simulink model "ThdRwRtStFwdBkwdCtrl"  (R2024b)
settings: Solver=FixedStepDiscrete  StartTime=0.0  StopTime=10.0  FixedStep=0.01  RelTol=1e-3
undefined symbols (not defined in the file or in its folder): KeSMSuMdMotFinshdTm_Val, KeSMSuMdRetryTm1_Val, KeSMSuModeReqDurgTm_Val
libraries: StCtrlLibBkRecln x1
settings Model: ModifiedHistory="2024.6.21 V2.1.0  557模式流程V1.6"  Creator=sn2xws  LastModifiedBy=sn55gm
settings SolverCC: AlgebraicLoopSolver=TrustRegion
settings DataIOCC: SaveFormat=StructureWithTime  ReturnWorkspaceOutputs=off
settings OptimizationCC: DefaultParameterBehavior=Inlined  EnhancedBackFolding=on  PassReuseOutputArgsAs=Individual arguments  ZeroExternalMemoryAtStartup=off  ZeroInternalMemoryAtStartup=off  OptimizeBlockOrder=speed  DifferentSizesBufferReuse=on  OptimizationCustomize=off  EfficientTunableParamExpr=on
settings DebuggingCC: ParameterTunabilityLossMsg=error  UnconnectedInputMsg=warning  UnconnectedOutputMsg=warning  UnconnectedLineMsg=warning  ArithmeticOperatorsInVariantConditions=warning
settings ModelReferenceCC: EnableRefExpFcnMdlSchedulingChecks=on  ModelReferenceNumInstancesAllowed=Single
settings SFSimCC: MATLABDynamicMemAlloc=off  CustomCodeUndefinedFunction=UseInterfaceOnly
settings RTWCC: Description=AUTOSAR  SystemTargetFile=autosar.tlc  GenCodeOnly=on  TemplateMakefile=ert_default_tmf  GenerateReport=on  IncludeHyperlinkInReport=on  LaunchReport=on  DataTypeReplacement=CDataTypesFixedWidth  GenerateTraceInfo=on  GenerateTraceReport=on  GenerateTraceReportSl=on  GenerateTraceReportSf=on  GenerateTraceReportEml=on  GPUComputeCapability=3.5
settings CodeAppCC: ForceParamTrailComments=on  IgnoreCustomStorageClasses=off  OperatorAnnotations=on  SimulinkDataObjDesc=on  SFDataObjDesc=on  InsertBlockDesc=on
settings STFCustomTargetCC: TargetLangStandard=C99 (ISO)  MultiwordLength=256  ParMdlRefBuildCompliant=on  CompOptLevelCompliant=on  IncludeMdlTerminateFcn=off  CombineOutputUpdateFcns=on  SuppressErrorStatus=on  ERTCustomFileBanners=on  SupportNonFinite=off  SupportComplex=off  SupportContinuousTime=off  SupportNonInlinedSFcns=off  RemoveResetFunc=on  MATLABClassNameForMDSCustomization=Simulink.SoftwareTarget.ERTCustomization  AutosarCompliant=on  UseToolchainInfoCompliant=on  LookupTableObjectStructAxisOrder=2,1,3,4,...  LUTObjectStructOrderEvenSpacing=Size,Table,Breakpoints  SystemTargetFile=autosar.tlc
settings ERTTargetCC: TargetLangStandard=C99 (ISO)  ConcurrentExecutionCompliant=off  IncludeMdlTerminateFcn=off  SuppressErrorStatus=on  SupportNonFinite=off  SupportComplex=off  ModelStepFunctionPrototypeControlCompliant=off  CPPClassGenCompliant=off  AutosarCompliant=on  LookupTableObjectStructAxisOrder=2,1,3,4,...  LUTObjectStructOrderEvenSpacing=Size,Table,Breakpoints  ERTCustomFileTemplate=example_file_process.tlc  ERTFilePackagingFormat=Compact  BooleanTrueId=TRUE  BooleanFalseId=FALSE  DynamicArrayContainerType=coder::array

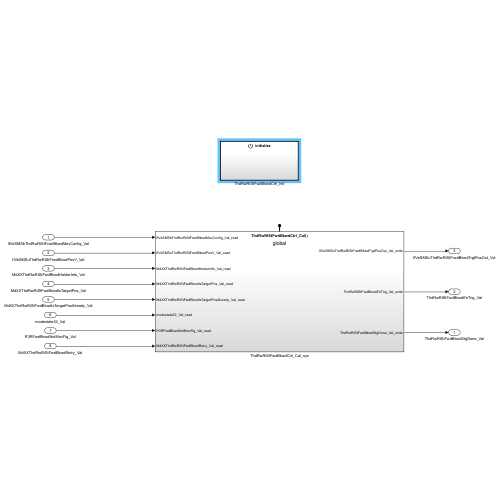
[thumbnail: Simulink's stored preview of the top-level diagram]
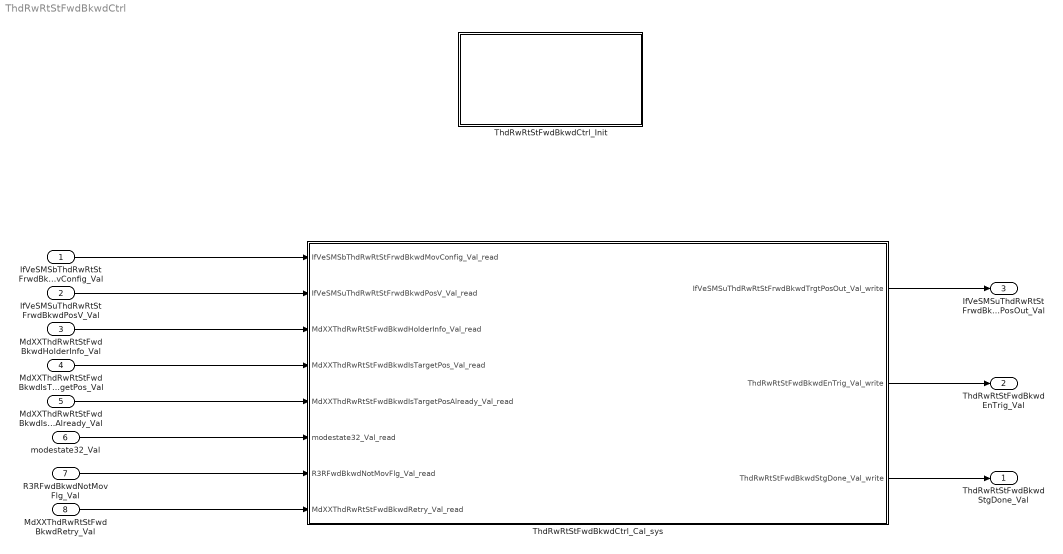
== system ThdRwRtStFwdBkwdCtrl ==
  IfVeSMSbThdRwRtStFrwdBkwdMovConfig_Val : Inport  OutDataTypeStr=boolean  PortDimensions=1
  IfVeSMSuThdRwRtStFrwdBkwdPosV_Val : Inport  Port=2  OutDataTypeStr=boolean  PortDimensions=1
  MdXXThdRwRtStFwdBkwdHolderInfo_Val : Inport  Port=3  OutDataTypeStr=uint32  PortDimensions=1
  MdXXThdRwRtStFwdBkwdIsTargetPos_Val : Inport  Port=4  OutDataTypeStr=uint32  PortDimensions=1
  MdXXThdRwRtStFwdBkwdIsTargetPosAlready_Val : Inport  Port=5  OutDataTypeStr=uint32  PortDimensions=1
  modestate32_Val : Inport  Port=6  OutDataTypeStr=uint32  PortDimensions=1
  R3RFwdBkwdNotMovFlg_Val : Inport  Port=7  OutDataTypeStr=boolean  PortDimensions=1
  MdXXThdRwRtStFwdBkwdRetry_Val : Inport  Port=8  OutDataTypeStr=uint32  PortDimensions=1
  ThdRwRtStFwdBkwdCtrl_Cal_sys : Subsystem
  ThdRwRtStFwdBkwdCtrl_Init : Subsystem
  ThdRwRtStFwdBkwdStgDone_Val : Outport  OutDataTypeStr=boolean  PortDimensions=1  VectorParamsAs1DForOutWhenUnconnected=off
  ThdRwRtStFwdBkwdEnTrig_Val : Outport  Port=2  OutDataTypeStr=boolean  PortDimensions=1  VectorParamsAs1DForOutWhenUnconnected=off
  IfVeSMSuThdRwRtStFrwdBkwdTrgtPosOut_Val : Outport  Port=3  OutDataTypeStr=boolean  PortDimensions=1  VectorParamsAs1DForOutWhenUnconnected=off
  wires:
  IfVeSMSbThdRwRtStFrwdBkwdMovConfig_Val/1 -> ThdRwRtStFwdBkwdCtrl_Cal_sys/1(IfVeSMSbThdRwRtStFrwdBkwdMovConfig_Val_read)
  IfVeSMSuThdRwRtStFrwdBkwdPosV_Val/1 -> ThdRwRtStFwdBkwdCtrl_Cal_sys/2(IfVeSMSuThdRwRtStFrwdBkwdPosV_Val_read)
  MdXXThdRwRtStFwdBkwdHolderInfo_Val/1 -> ThdRwRtStFwdBkwdCtrl_Cal_sys/3(MdXXThdRwRtStFwdBkwdHolderInfo_Val_read)
  MdXXThdRwRtStFwdBkwdIsTargetPos_Val/1 -> ThdRwRtStFwdBkwdCtrl_Cal_sys/4(MdXXThdRwRtStFwdBkwdIsTargetPos_Val_read)
  MdXXThdRwRtStFwdBkwdIsTargetPosAlready_Val/1 -> ThdRwRtStFwdBkwdCtrl_Cal_sys/5(MdXXThdRwRtStFwdBkwdIsTargetPosAlready_Val_read)
  modestate32_Val/1 -> ThdRwRtStFwdBkwdCtrl_Cal_sys/6(modestate32_Val_read)
  R3RFwdBkwdNotMovFlg_Val/1 -> ThdRwRtStFwdBkwdCtrl_Cal_sys/7(R3RFwdBkwdNotMovFlg_Val_read)
  ThdRwRtStFwdBkwdCtrl_Cal_sys/1(IfVeSMSuThdRwRtStFrwdBkwdTrgtPosOut_Val_write) -> IfVeSMSuThdRwRtStFrwdBkwdTrgtPosOut_Val/1
  ThdRwRtStFwdBkwdCtrl_Cal_sys/2(ThdRwRtStFwdBkwdEnTrig_Val_write) -> ThdRwRtStFwdBkwdEnTrig_Val/1
  ThdRwRtStFwdBkwdCtrl_Cal_sys/3(ThdRwRtStFwdBkwdStgDone_Val_write) -> ThdRwRtStFwdBkwdStgDone_Val/1
  MdXXThdRwRtStFwdBkwdRetry_Val/1 -> ThdRwRtStFwdBkwdCtrl_Cal_sys/8(MdXXThdRwRtStFwdBkwdRetry_Val_read)

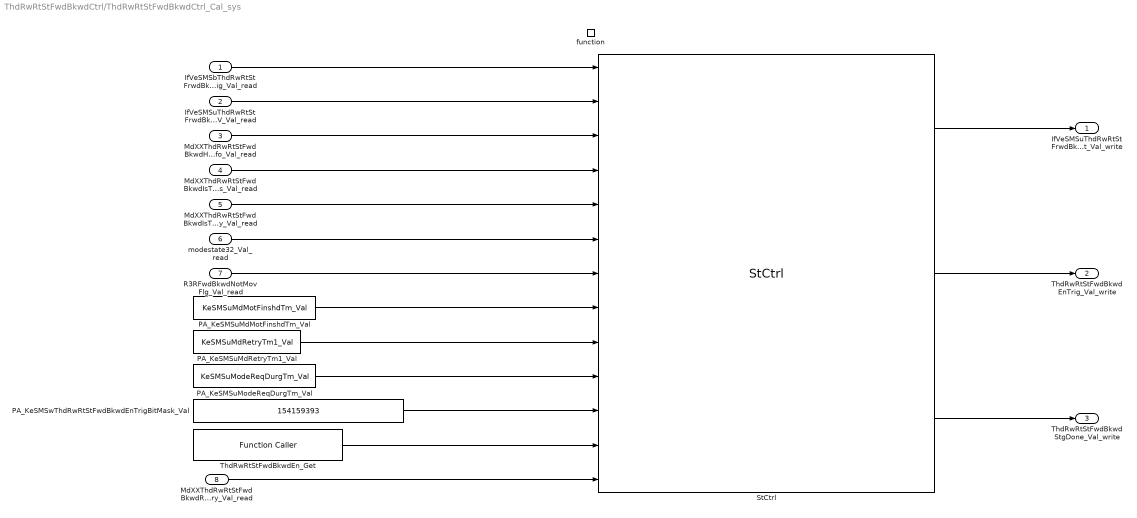
== system ThdRwRtStFwdBkwdCtrl/ThdRwRtStFwdBkwdCtrl_Cal_sys ==
  IfVeSMSbThdRwRtStFrwdBkwdMovConfig_Val_read : Inport
  IfVeSMSuThdRwRtStFrwdBkwdPosV_Val_read : Inport  Port=2
  MdXXThdRwRtStFwdBkwdHolderInfo_Val_read : Inport  Port=3
  MdXXThdRwRtStFwdBkwdIsTargetPos_Val_read : Inport  Port=4
  MdXXThdRwRtStFwdBkwdIsTargetPosAlready_Val_read : Inport  Port=5
  modestate32_Val_read : Inport  Port=6
  R3RFwdBkwdNotMovFlg_Val_read : Inport  Port=7
  MdXXThdRwRtStFwdBkwdRetry_Val_read : Inport  Port=8
  function : TriggerPort  TriggerType=function-call  IsSimulinkFunction=on  FunctionName=ThdRwRtStFwdBkwdCtrl_Cal  VariantControl=(inherit)
  PA_KeSMSuMdMotFinshdTm_Val : Constant  Value=KeSMSuMdMotFinshdTm_Val
  PA_KeSMSuMdRetryTm1_Val : Constant  Value=KeSMSuMdRetryTm1_Val
  PA_KeSMSuModeReqDurgTm_Val : Constant  Value=KeSMSuModeReqDurgTm_Val
  PA_KeSMSwThdRwRtStFwdBkwdEnTrigBitMask_Val : Constant  Value=154159393  OutDataTypeStr=uint32
  StCtrl : StCtrlLibBkRecln/StCtrl  SystemSampleTime=-1  VariantActivationTime=update diagram  AllowFlexibleInterface=on  Latency=0  AutoFrameSizeCalculation=off
  ThdRwRtStFwdBkwdEn_Get : FunctionCaller  FunctionPrototype=data = ThdRwRtStFwdBkwdEn_Get()  InputArgumentSpecifications=<Enter example>  OutputArgumentSpecifications=uint32(1)
  IfVeSMSuThdRwRtStFrwdBkwdTrgtPosOut_Val_write : Outport  VectorParamsAs1DForOutWhenUnconnected=off
      settings: EnsureOutportIsVirtual=on
  ThdRwRtStFwdBkwdEnTrig_Val_write : Outport  Port=2  VectorParamsAs1DForOutWhenUnconnected=off
      settings: EnsureOutportIsVirtual=on
  ThdRwRtStFwdBkwdStgDone_Val_write : Outport  Port=3  VectorParamsAs1DForOutWhenUnconnected=off
      settings: EnsureOutportIsVirtual=on
  wires:
  StCtrl/1 -> IfVeSMSuThdRwRtStFrwdBkwdTrgtPosOut_Val_write/1
  StCtrl/2 -> ThdRwRtStFwdBkwdEnTrig_Val_write/1
  StCtrl/3 -> ThdRwRtStFwdBkwdStgDone_Val_write/1
  modestate32_Val_read/1 -> StCtrl/6
  R3RFwdBkwdNotMovFlg_Val_read/1 -> StCtrl/7
  MdXXThdRwRtStFwdBkwdIsTargetPosAlready_Val_read/1 -> StCtrl/5
  MdXXThdRwRtStFwdBkwdIsTargetPos_Val_read/1 -> StCtrl/4
  MdXXThdRwRtStFwdBkwdHolderInfo_Val_read/1 -> StCtrl/3
  IfVeSMSuThdRwRtStFrwdBkwdPosV_Val_read/1 -> StCtrl/2
  IfVeSMSbThdRwRtStFrwdBkwdMovConfig_Val_read/1 -> StCtrl/1
  PA_KeSMSwThdRwRtStFwdBkwdEnTrigBitMask_Val/1 -> StCtrl/11
  ThdRwRtStFwdBkwdEn_Get/1 -> StCtrl/12
  PA_KeSMSuMdMotFinshdTm_Val/1 -> StCtrl/8
  PA_KeSMSuModeReqDurgTm_Val/1 -> StCtrl/10
  PA_KeSMSuMdRetryTm1_Val/1 -> StCtrl/9
  MdXXThdRwRtStFwdBkwdRetry_Val_read/1 -> StCtrl/13

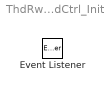
== system ThdRwRtStFwdBkwdCtrl/ThdRwRtStFwdBkwdCtrl_Init ==
  Event Listener : EventListener  EventName=reset
